simulink model "PCCI_2"  (R2024b)
settings: Solver=FixedStepDiscrete  StartTime=0.0  StopTime=1  FixedStep=0.001  RelTol=1e-3
settings Model: Creator=LENOVO  LastModifiedBy=LENOVO
settings OptimizationCC: DefaultParameterBehavior=Inlined  EnhancedBackFolding=on  PassReuseOutputArgsAs=Individual arguments  ZeroExternalMemoryAtStartup=off  ZeroInternalMemoryAtStartup=off  OptimizeBlockOrder=speed  DifferentSizesBufferReuse=on  OptimizationCustomize=off  EfficientTunableParamExpr=on
settings DebuggingCC: ParameterTunabilityLossMsg=error
settings SFSimCC: MATLABDynamicMemAlloc=off
settings RTWCC: Description=Embedded Coder  SystemTargetFile=ert.tlc  GenCodeOnly=on  TemplateMakefile=ert_default_tmf  GenerateReport=on  LaunchReport=on  GenerateCodeMetricsReport=on
settings CodeAppCC: ForceParamTrailComments=on  IgnoreCustomStorageClasses=off  OperatorAnnotations=on  SimulinkDataObjDesc=on  SFDataObjDesc=on  InsertBlockDesc=on
settings ERTTargetCC: TargetLangStandard=C99 (ISO)  GenerateSampleERTMain=on  ERTCustomFileTemplate=example_file_process.tlc

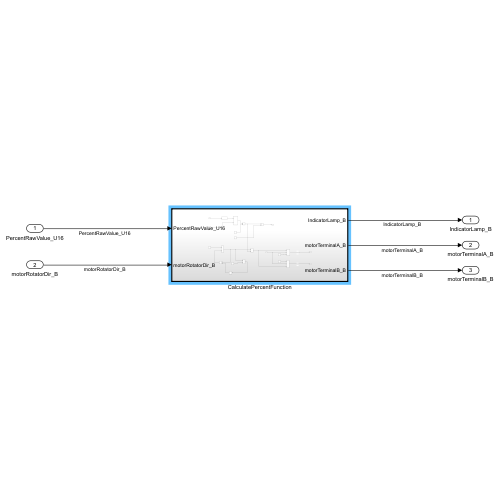
[thumbnail: Simulink's stored preview of the top-level diagram]
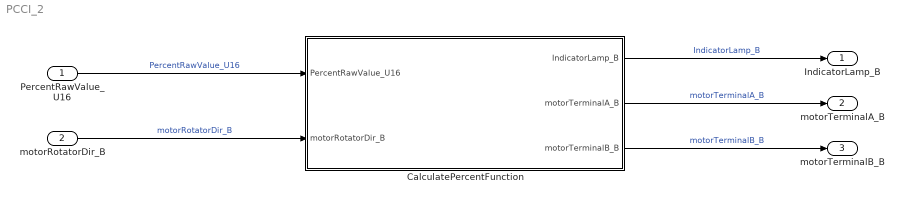
== system PCCI_2 ==
  PercentRawValue_U16 : Inport
  motorRotatorDir_B : Inport  Port=2
  CalculatePercentFunction : Subsystem  TreatAsAtomicUnit=on
      settings: RTWFcnNameOpts=Use subsystem name  RTWFileNameOpts=Use subsystem name
  IndicatorLamp_B : Outport  OutDataTypeStr=boolean
  motorTerminalA_B : Outport  Port=2  OutDataTypeStr=boolean
  motorTerminalB_B : Outport  Port=3  OutDataTypeStr=boolean
  wires:
  PercentRawValue_U16/1 -> CalculatePercentFunction/1(PercentRawValue_U16)  "PercentRawValue_U16"
  CalculatePercentFunction/1(IndicatorLamp_B) -> IndicatorLamp_B/1  "IndicatorLamp_B"
  motorRotatorDir_B/1 -> CalculatePercentFunction/2(motorRotatorDir_B)  "motorRotatorDir_B"
  CalculatePercentFunction/3(motorTerminalB_B) -> motorTerminalB_B/1  "motorTerminalB_B"
  CalculatePercentFunction/2(motorTerminalA_B) -> motorTerminalA_B/1  "motorTerminalA_B"

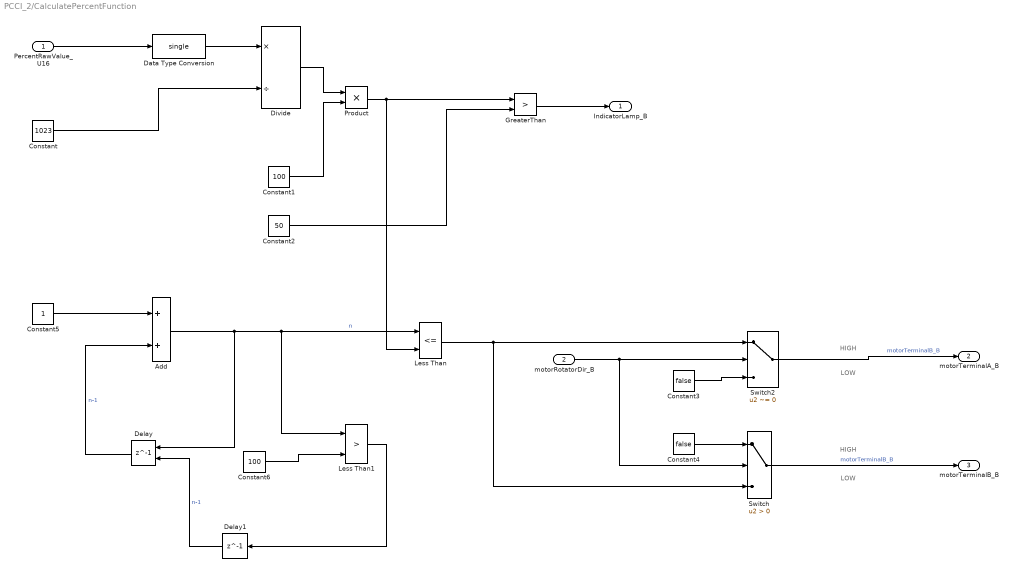
== system PCCI_2/CalculatePercentFunction ==
  note: HIGH
  note: HIGH
  note: LOW
  note: LOW
  PercentRawValue_U16 : Inport
  motorRotatorDir_B : Inport  Port=2
  Add : Sum
  Constant : Constant  Value=1023  OutDataTypeStr=single
  Constant1 : Constant  Value=100  OutDataTypeStr=uint8
  Constant2 : Constant  Value=50  OutDataTypeStr=uint8
  Constant3 : Constant  Value=false  OutDataTypeStr=boolean
  Constant4 : Constant  Value=false  OutDataTypeStr=boolean
  Constant5 : Constant  OutDataTypeStr=uint8
  Constant6 : Constant  Value=100  OutDataTypeStr=uint8
  Data Type Conversion : DataTypeConversion  OutDataTypeStr=single  SaturateOnIntegerOverflow=off  RndMeth=Floor
  Delay : Delay  DelayLength=1  ExternalReset=Rising
      settings: InputPortMap=u0,r5
  Delay1 : Delay  DelayLength=1
  Divide : Product  Inputs=*/
  GreaterThan : RelationalOperator  Operator=>  OutDataTypeStr=boolean  RndMeth=Simplest  InputSameDT=off
  Less Than : RelationalOperator  Operator=<=  OutDataTypeStr=boolean  RndMeth=Simplest  InputSameDT=off
  Less Than1 : RelationalOperator  Operator=>  OutDataTypeStr=boolean  RndMeth=Simplest  InputSameDT=off
  Product : Product
  Switch : Switch  Criteria=u2 > Threshold  SaturateOnIntegerOverflow=off  InputSameDT=off
  Switch2 : Switch  Criteria=u2 ~= 0  SaturateOnIntegerOverflow=off  InputSameDT=off
  IndicatorLamp_B : Outport  OutDataTypeStr=boolean
  motorTerminalA_B : Outport  Port=2  OutDataTypeStr=boolean
  motorTerminalB_B : Outport  Port=3  OutDataTypeStr=boolean
  wires:
  PercentRawValue_U16/1 -> Data Type Conversion/1
  Constant/1 -> Divide/2
  Data Type Conversion/1 -> Divide/1
  Divide/1 -> Product/1
  Constant1/1 -> Product/2
  Constant2/1 -> GreaterThan/2
  GreaterThan/1 -> IndicatorLamp_B/1
  Switch/1 -> motorTerminalB_B/1  "motorTerminalB_B"
  Switch2/1 -> motorTerminalA_B/1  "motorTerminalB_B"
  motorRotatorDir_B/1 -> Switch/2, Switch2/2
  Constant4/1 -> Switch/1
  Constant5/1 -> Add/1
  Add/1 -> Delay/1, Less Than1/1, Less Than/1  "n"
  Delay/1 -> Add/2  "n-1"
  Constant6/1 -> Less Than1/2
  Less Than1/1 -> Delay1/1
  Delay1/1 -> Delay/2  "n-1"
  Product/1 -> Less Than/2, GreaterThan/1
  Constant3/1 -> Switch2/3
  Less Than/1 -> Switch/3, Switch2/1
